simulink model "Lotka_Volterra_v1"  (R2024a)
settings: Solver=ode4  StartTime=0.0  StopTime=200  FixedStep=.01  RelTol=1e-3
model workspace (MATLAB code in the model file):
  | % Parámetros del modelo
  | lambda1 = 1;   % Tasa natural de nacimiento de los predadores
  | lambda2 = 2;   % Tasa natural de nacimiento de las presas
  | gamma1 = 2;    % Tasa de mortalidad de los depredadores
  | gamma2 = 1;    % Tasa de mortalidad de las presas
  | alpha1 = 2;    % Tasa de la eficiencia de conversión de presas en nuevos depredadores.
  | alpha2 = 2;    % Tasa de encuentro entre presas y depredadores
  | 
  | % Condiciones iniciales
  | N1 = 10;  % Población inicial de depredadores
  | N2 = 20;   % Población inicial de presas
  | x0 = [N1; N2];
settings Model: Creator=scpmoxxa  LastModifiedBy=scpmoxxa
settings OptimizationCC: ReuseModelBlockBuffer=off
settings RTWCC: GPUComputeCapability=3.5

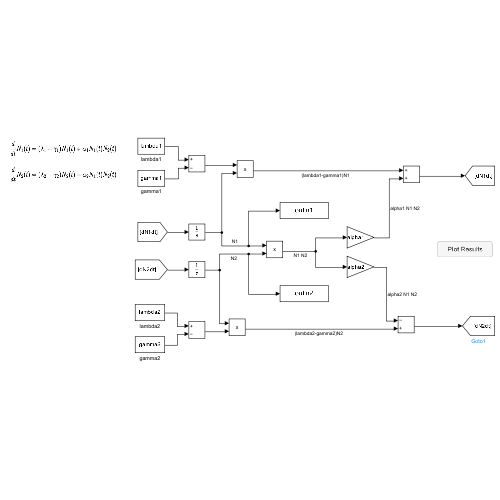
[thumbnail: Simulink's stored preview of the top-level diagram]
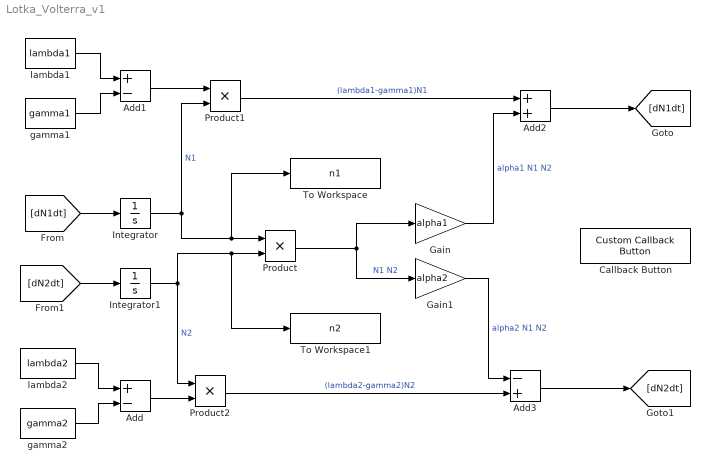
== system Lotka_Volterra_v1 ==
  Add : Sum  Inputs=+-
  Add1 : Sum  Inputs=+-
  Add2 : Sum
  Add3 : Sum  Inputs=-+
  Callback Button : CustomCallbackButton  Configuration="{\"components\":[{\"name\":\"BackgroundImageComponent\",\"settings\":{\"image\":{\"size\":[0,0],\"src\":\"default\",\"srcOrientation\":\"Right\"},\"position\":[0,0,1,1]}},{\"name\":\"ButtonStateComponent\",\"settings\":{\"buttonType\":\"momentary\",\"clickFcn\":\"close all\\nt = out.tout;\\nx = [out.n1, out.n2];\\n\\n% Gr�fico de las poblaciones de presas y depredadores\\nfigure;\\nsubplot(121)\\nplot(t, x(:,1), 'b', 'LineWidth', 2); hold on;\\nplot(t, x(:,2), 'r', 'LineWidth', 2);\\nxlabel('Tiempo');\\nylabel('Poblaci�n');\\ntitle('Din�mica de las poblaciones de presas y depredadores');\\nlegend('Presas', 'Depredadores');\\ngrid on;\\nsubplot(122)\\nplot(x(:,1),x(:,2));\\nxlabel('N1');ylabel('N2')\",\"onValue\":1,\"position\":[0,0,1,1],\"pressDelay\":\"500\",\"pressFcn\":\"\",\"repeatInterval\":\"0\",\"states\":[{\"horizontalAlignment\":\"center\",\"image\":{\"position\":[0,0,1,1],\"src\":\"default\",\"srcOrientation\":\"Right\"},\"label\":{\"color\":[0.01176470588,0.01176470588,0.01176470588,1],\"icon\":{\"size\":[0,0],\"src\":\"default\",\"srcOrientation\":\"Right\"},\"iconPlacement\":\"left\",\"text\":{\"content\":\"Plot Results\"}},\"labelOffset\":[0,0],\"verticalAlignment\":\"middle\"},{\"horizontalAlignment\":\"center\",\"image\":{\"position\":[0,0,1,1],\"src\":\"default\",\"srcOrientation\":\"Right\"},\"label\":{\"color\":[0.01176470588,0.01176470588,0.01176470588,1],\"icon\":{\"size\":[0,0],\"src\":\"default\",\"srcOrientation\":\"Right\"},\"iconPlacement\":\"left\",\"text\":{\"content\":\"Plot Results\"}},\"labelOffset\":[0,0],\"verticalAlignment\":\"middle\"},{\"horizontalAlignment\":\"center\",\"image\":{\"position\":[0,0,1,1],\"src\":\"default\",\"srcOrientation\":\"Right\"},\"label\":{\"color\":[0.01176470588,0.01176470588,0.01176470588,1],\"icon\":{\"size\":[0,0],\"src\":\"default\",\"srcOrientation\":\"Right\"},\"iconPlacement\":\"left\",\"text\":{\"content\":\"Plot Results\"}},\"labelOffset\":[0,0],\"verticalAlignment\":\"middle\"},{\"horizontalAlignment\":\"center\",\"image\":{\"position\":[0,0,1,1],\"src\":\"default\",\"srcOrientation\":\"Right\"},\"label\":{\"color\":[0.01176470588,0.01176470588,0.01176470588,1],\"icon\":{\"size\":[0,0],\"src\":\"default\",\"srcOrientation\":\"Right\"},\"iconPlacement\":\"left\",\"text\":{\"content\":\"Plot Results\"}},\"labelOffset\":[0,0],\"verticalAlignment\":\"middle\"}]}},{\"name\":\"ForegroundImageComponent\",\"settings\":{\"image\":{\"size\":[0,0],\"src\":\"default\",\"srcOrientation\":\"Right\"},\"isForeground\":1,\"position\":[0,0,1,1]}}],\"settings\":{\"BindingType\":\"standalone\",\"backgroundColor\":[244,244,244,1],\"backgroundOffset\":0.2,\"backgroundOpacity\":1,\"fixedAspectRatio\":\"off\",\"foregroundColor\":[0.01176470588,0.01176470588,0.01176470588,1],\"migratedFromLegacy\":true,\"useBackgroundColor\":true,\"variant\":\"callback\",\"version\":\"R2023a\"},\"type\":\"Button\"}"  CustomBackgroundColor="{\"color\":[0.9568627451,0.9568627451,0.9568627451],\"show\":true}"
  Gain : Gain  Gain=alpha1
  Gain1 : Gain  Gain=alpha2
  Integrator : Integrator  InitialCondition=N1
  Integrator1 : Integrator  InitialCondition=N2
  Product : Product
  Product1 : Product
  Product2 : Product
  To Workspace : ToWorkspace  VariableName=n1  SampleTime=-1
  To Workspace1 : ToWorkspace  VariableName=n2  SampleTime=-1
  gamma1 : Constant  Value=gamma1
  gamma2 : Constant  Value=gamma2
  lambda1 : Constant  Value=lambda1
  lambda2 : Constant  Value=lambda2
  wires:
  Integrator/1 -> To Workspace/1, Product/1, Product1/2  "N1"
  Integrator1/1 -> Product2/1, To Workspace1/1, Product/2  "N2"
  Product/1 -> Gain/1, Gain1/1  "N1 N2"
  gamma2/1 -> Add/2
  lambda2/1 -> Add/1
  gamma1/1 -> Add1/2
  lambda1/1 -> Add1/1
  Add1/1 -> Product1/1
  Add/1 -> Product2/2
  Product1/1 -> Add2/1  "(lambda1-gamma1)N1"
  Gain/1 -> Add2/2  "alpha1 N1 N2"
  Add2/1 -> [dN1dt]
  [dN1dt] -> Integrator/1
  Product2/1 -> Add3/2  "(lambda2-gamma2)N2"
  Gain1/1 -> Add3/1  "alpha2 N1 N2"
  Add3/1 -> [dN2dt]
  [dN2dt] -> Integrator1/1
